simulink model "martin_arbot_v2offset"  (R2020a)
settings: Solver=ode15s  StartTime=0.0  StopTime=15  MaxStep=.01  RelTol=1e-3  AbsTol=1e-4
InitFcn:
  | % currentFolder = pwd;
  | % parent = '../Targeting';
  | % environment = '../Environment';
  | % addpath(genpath(parent));
  | % addpath(genpath(environment));
  | 
  | startup_ARbot;
  | chute2_DataFile;
  | guard_DataFile1;
  | shelf_DataFile1;
  | bin_assembly_DataFile;
values from neighbouring files (symbols this model uses):
  Environment = append(cwd,'/Environment')    [init_root_paths_mac.m]    (also in init_root_paths_windows.m = append(cwd,'\Environment'))
undefined symbols (not defined in the file or in its folder): belt_h, belt_l, belt_spd, belt_w, box1_dim, box2_dim, box3_dim, box4_dim, box5_dim, cube_d, deposit_joint_angle, Extr_Data_LinkHoles, floor_d, floor_l, ikSol, initial_joints, m, n, P_C, safe_via_angles, sigbuilder_block, smiData, X, Y, Z
libraries: sm_lib x145, nesl_utility x78, Contact_Forces_Lib x10, simulink x5, Parts_Lib x5, dspsrcs4 x1
(part 1 of 5)
settings Model: Creator=logan  LastModifiedBy=mcontr
settings SFSimCC: CustomCodeUndefinedFunction=UseInterfaceOnly
settings DiagnosticsConfigSet: SimMechanicsConflictingReferenceFrames=none  SimMechanicsRigidlyBoundBlock=warning

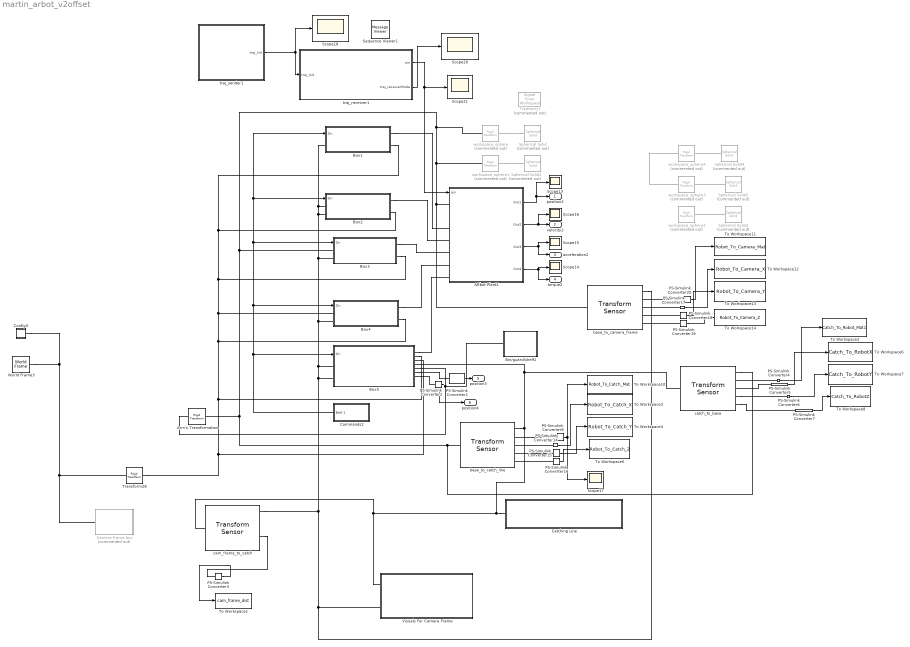
== system martin_arbot_v2offset ==
  ARbot Plant1 : Subsystem
  Arm's Transformation : sm_lib/Frames and Transforms/Rigid Transform  TranslationMethod=Cartesian  TranslationStandardOffset=10  TranslationLengthUnit=m  TranslationStandardAxis=+Y  TranslationCartesianOffset=box_xyz_pos_offset  TranslationROffset=0  TranslationROffsetUnits=m  TranslationZOffset=0  TranslationZOffsetUnits=m  TranslationThetaOffset=0  TranslationThetaOffsetUnits=deg  RotationMethod=RotationSequence  RotationAngleUnits=deg  RotationStandardAxis=+Z  RotationAngle=270  RotationArbitraryAxis=smiData.RigidTransform(1).axis  FollAlignAxisA=+X  BaseAlignAxisA=+Y  FollAlignAxisB=+Y  BaseAlignAxisB=+Z  RotationSequenceAxes=FollowerAxes  RotationSequence=XYZ  RotationSequenceAngles=box_xyz_angle_offset  RotationSequenceAnglesUnits=deg  RotationMatrix=[1 0 0; 0 1 0; 0 0 1]
  Bin/guard/shelf1 : Subsystem
  Box1 : Subsystem
  Box2 : Subsystem
  Box3 : Subsystem
  Box4 : Subsystem
  Box5 : Subsystem
  Camera frame box : Subsystem  Commented=on
  Catching Line : Subsystem
  Commands2 : Subsystem  Tag=STV Subsys  LoadFcn=sigbuilder_block('load');  StartFcn=sigbuilder_block('start');  StopFcn=sigbuilder_block('stop');  ClipboardFcn=sigbuilder_block('clipboard');  mask(Sigbuilder block){tuvar=[0:10]}
      mask help: Simulink:masks:SigbuilderBlock_MD
      mask init:
      | if ~strcmp(get_param(bdroot(gcbh),'SimulationStatus'),'stopped') tuvar = sigbuilder_block('maskInit'); end
      settings: CopyFcn=sigbuilder_block('copy');  DeleteFcn=sigbuilder_block('delete');  ModelCloseFcn=sigbuilder_block('modelClose');  PreSaveFcn=sigbuilder_block('preSave');  PauseFcn=sigbuilder_block('pause');  ContinueFcn=sigbuilder_block('continue');  NameChangeFcn=sigbuilder_block('namechange');  OpenFcn=sigbuilder_block('open',[107 163.5 543 316.5 ]);  CloseFcn=sigbuilder_block('close');
      mask Display: plot(0, 0, 100, 100,[2, 2, 32, 32, 2], [68, 8, 8, 68, 68],[32, 2], [38, 38], [32, 19, 2],[53, 60, 44], [32, 17, 17, 2],[16, 16, 31, 31]);txt = getActiveGroup(gcbh);text(2, 100, txt,'verticalAlignment', 'top');
  Config3 : Subsystem
  PS-Simulink Converter{1..7,9,14..20} (15 alike) : nesl_utility/PS-Simulink Converter  PhysicalDomain=network_engine_domain  SubClassName=ps_output  LeftPortType=input  RightPortType=output  PseudoPeriodic=off  Frequencies=[]  Unit=inherit  AffineConversion=off
  Scope{13..18,20..21} (8 alike) : Scope
  Sequence Viewer1 : MessageViewer
  Spherical Solid : sm_lib/Body Elements/Spherical Solid  Commented=on  GraphicAmbientColor=[0.15 0.15 0.15 1.0]  BasedOnType=Density  CenterOfMass=[0 0 0]  CenterOfMassUnits=m  GraphicDiffuseColor=[1.0 0.6 0.2]  Density=1000  DensityUnits=kg/m^3  DoExposeReferenceFrame=on  GraphicEmissiveColor=[0.0 0.0 0.0 1.0]  ExportEntireGeometry=off  SerializedExposedGeometries=<ExposedGeometries/>  SerializedFrames=<Frames/>  MarkerShape=Sphere  MarkerSize=10  GraphicType=FromGeometry  InertiaType=CalculateFromGeometry  Mass=1  MassUnits=kg  MomentsOfInertia=[1 1 1]  MomentsOfInertiaUnits=kg*m^2  GraphicOpacity=1.0  ProductsOfInertia=[0 0 0]  ProductsOfInertiaUnits=kg*m^2  GraphicShininess=75  GraphicSpecularColor=[0.5 0.5 0.5 1.0]  SphereRadius=0.05  SphereRadiusUnits=m  GraphicVisPropType=SimpleVisualProperties
  Spherical Solid1 : sm_lib/Body Elements/Spherical Solid  Commented=on  GraphicAmbientColor=[0.15 0.15 0.15 1.0]  BasedOnType=Density  CenterOfMass=[0 0 0]  CenterOfMassUnits=m  GraphicDiffuseColor=[1.0 0.6 0.2]  Density=1000  DensityUnits=kg/m^3  DoExposeReferenceFrame=on  GraphicEmissiveColor=[0.0 0.0 0.0 1.0]  ExportEntireGeometry=off  SerializedExposedGeometries=<ExposedGeometries/>  SerializedFrames=<Frames/>  MarkerShape=Sphere  MarkerSize=10  GraphicType=FromGeometry  InertiaType=CalculateFromGeometry  Mass=1  MassUnits=kg  MomentsOfInertia=[1 1 1]  MomentsOfInertiaUnits=kg*m^2  GraphicOpacity=1.0  ProductsOfInertia=[0 0 0]  ProductsOfInertiaUnits=kg*m^2  GraphicShininess=75  GraphicSpecularColor=[0.5 0.5 0.5 1.0]  SphereRadius=0.05  SphereRadiusUnits=m  GraphicVisPropType=SimpleVisualProperties
  Spherical Solid2 : sm_lib/Body Elements/Spherical Solid  Commented=on  GraphicAmbientColor=[0.15 0.15 0.15 1.0]  BasedOnType=Density  CenterOfMass=[0 0 0]  CenterOfMassUnits=m  GraphicDiffuseColor=[0.0 0.8 0.4]  Density=1000  DensityUnits=kg/m^3  DoExposeReferenceFrame=on  GraphicEmissiveColor=[0.0 0.0 0.0 1.0]  ExportEntireGeometry=off  SerializedExposedGeometries=<ExposedGeometries/>  SerializedFrames=<Frames/>  MarkerShape=Sphere  MarkerSize=10  GraphicType=FromGeometry  InertiaType=CalculateFromGeometry  Mass=1  MassUnits=kg  MomentsOfInertia=[1 1 1]  MomentsOfInertiaUnits=kg*m^2  GraphicOpacity=1.0  ProductsOfInertia=[0 0 0]  ProductsOfInertiaUnits=kg*m^2  GraphicShininess=75  GraphicSpecularColor=[0.5 0.5 0.5 1.0]  SphereRadius=0.05  SphereRadiusUnits=m  GraphicVisPropType=SimpleVisualProperties
  Spherical Solid3 : sm_lib/Body Elements/Spherical Solid  Commented=on  GraphicAmbientColor=[0.15 0.15 0.15 1.0]  BasedOnType=Density  CenterOfMass=[0 0 0]  CenterOfMassUnits=m  GraphicDiffuseColor=[0.0 0.8 0.4]  Density=1000  DensityUnits=kg/m^3  DoExposeReferenceFrame=on  GraphicEmissiveColor=[0.0 0.0 0.0 1.0]  ExportEntireGeometry=off  SerializedExposedGeometries=<ExposedGeometries/>  SerializedFrames=<Frames/>  MarkerShape=Sphere  MarkerSize=10  GraphicType=FromGeometry  InertiaType=CalculateFromGeometry  Mass=1  MassUnits=kg  MomentsOfInertia=[1 1 1]  MomentsOfInertiaUnits=kg*m^2  GraphicOpacity=1.0  ProductsOfInertia=[0 0 0]  ProductsOfInertiaUnits=kg*m^2  GraphicShininess=75  GraphicSpecularColor=[0.5 0.5 0.5 1.0]  SphereRadius=0.05  SphereRadiusUnits=m  GraphicVisPropType=SimpleVisualProperties
  Spherical Solid4 : sm_lib/Body Elements/Spherical Solid  Commented=on  GraphicAmbientColor=[0.15 0.15 0.15 1.0]  BasedOnType=Density  CenterOfMass=[0 0 0]  CenterOfMassUnits=m  GraphicDiffuseColor=[0.0 0.8 0.4]  Density=1000  DensityUnits=kg/m^3  DoExposeReferenceFrame=on  GraphicEmissiveColor=[0.0 0.0 0.0 1.0]  ExportEntireGeometry=off  SerializedExposedGeometries=<ExposedGeometries/>  SerializedFrames=<Frames/>  MarkerShape=Sphere  MarkerSize=10  GraphicType=FromGeometry  InertiaType=CalculateFromGeometry  Mass=1  MassUnits=kg  MomentsOfInertia=[1 1 1]  MomentsOfInertiaUnits=kg*m^2  GraphicOpacity=1.0  ProductsOfInertia=[0 0 0]  ProductsOfInertiaUnits=kg*m^2  GraphicShininess=75  GraphicSpecularColor=[0.5 0.5 0.5 1.0]  SphereRadius=0.05  SphereRadiusUnits=m  GraphicVisPropType=SimpleVisualProperties
  To Workspace1 : ToWorkspace  VariableName=cam_frame_dist  SampleTime=-1
      settings: Save2DSignal=2-D array (concatenate along first dimension)
  To Workspace10 : ToWorkspace  VariableName=Robot_To_Catch_Mat  SampleTime=-1
      settings: Save2DSignal=2-D array (concatenate along first dimension)
  To Workspace11 : ToWorkspace  VariableName=Robot_To_Camera_Mat  SampleTime=-1
      settings: Save2DSignal=2-D array (concatenate along first dimension)
  To Workspace12 : ToWorkspace  VariableName=Robot_To_Camera_X  SampleTime=-1
      settings: Save2DSignal=2-D array (concatenate along first dimension)
  To Workspace13 : ToWorkspace  VariableName=Robot_To_Camera_Y  SampleTime=-1
      settings: Save2DSignal=2-D array (concatenate along first dimension)
  To Workspace14 : ToWorkspace  VariableName=Robot_To_Camera_Z  SampleTime=-1
      settings: Save2DSignal=2-D array (concatenate along first dimension)
  To Workspace2 : ToWorkspace  VariableName=Catch_To_Robot_Mat1  SampleTime=-1
      settings: Save2DSignal=2-D array (concatenate along first dimension)
  To Workspace3 : ToWorkspace  VariableName=Robot_To_Catch_X  SampleTime=-1
      settings: Save2DSignal=2-D array (concatenate along first dimension)
  To Workspace4 : ToWorkspace  VariableName=Robot_To_Catch_Y  SampleTime=-1
      settings: Save2DSignal=2-D array (concatenate along first dimension)
  To Workspace5 : ToWorkspace  VariableName=Robot_To_Catch_Z  SampleTime=-1
      settings: Save2DSignal=2-D array (concatenate along first dimension)
  To Workspace6 : ToWorkspace  VariableName=Catch_To_RobotX  SampleTime=-1
      settings: Save2DSignal=2-D array (concatenate along first dimension)
  To Workspace7 : ToWorkspace  VariableName=Catch_To_RobotY  SampleTime=-1
      settings: Save2DSignal=2-D array (concatenate along first dimension)
  To Workspace8 : ToWorkspace  VariableName=Catch_To_RobotZ  SampleTime=-1
      settings: Save2DSignal=2-D array (concatenate along first dimension)
  Trajectory1 : dspsrcs4/Signal From Workspace  Commented=on  X=th  Ts=.08  nsamps=1  OutputAfterFinalValue=Holding final value  ignoreOrWarnInputAndFrameLengths=off  OutputFrames=off
  Transform28 : sm_lib/Frames and Transforms/Rigid Transform  TranslationMethod=Cartesian  TranslationStandardOffset=10  TranslationLengthUnit=m  TranslationStandardAxis=+Y  TranslationCartesianOffset=belt_pos_offset  TranslationROffset=0  TranslationROffsetUnits=m  TranslationZOffset=0  TranslationZOffsetUnits=m  TranslationThetaOffset=0  TranslationThetaOffsetUnits=deg  RotationMethod=RotationSequence  RotationAngleUnits=deg  RotationStandardAxis=+Z  RotationAngle=90  RotationArbitraryAxis=smiData.RigidTransform(1).axis  FollAlignAxisA=+X  BaseAlignAxisA=+Y  FollAlignAxisB=+Y  BaseAlignAxisB=+Z  RotationSequenceAxes=BaseAxes  RotationSequence=XYZ  RotationSequenceAngles=belt_angle_offset  RotationSequenceAnglesUnits=deg  RotationMatrix=[1 0 0; 0 1 0; 0 0 1]
  Visuals For Camera Frame : Subsystem
  World Frame3 : sm_lib/Frames and Transforms/World Frame
  base_to_camera_frame : sm_lib/Frames and Transforms/Transform Sensor  MeasurementFrame=Base  SenseAngle=off  SenseAxis=off  SenseAngle1=off  SenseAngle2=off  SenseAngle3=off  SenseQ=off  SenseR=on  SenseOmegaX=off  SenseOmegaY=off  SenseOmegaZ=off  SenseOmega1=off  SenseOmega2=off  SenseOmega3=off  SenseQDot=off  SenseRDot=off  SenseAlphaX=off  SenseAlphaY=off  SenseAlphaZ=off  SenseAlpha1=off  SenseAlpha2=off  SenseAlpha3=off  SenseQDDot=off  SenseRDDot=off  SenseX=on  SenseY=on  SenseZ=on  SenseRad=off  SenseAzim=off  SenseDist=off  SenseInc=off  SenseXDot=off  SenseYDot=off  SenseZDot=off  SenseRadDot=off  SenseAzimDot=off  SenseDistDot=off  SenseIncDot=off  SenseXDDot=off  SenseYDDot=off  SenseZDDot=off  SenseRadDDot=off  SenseAzimDDot=off  SenseDistDDot=off  SenseIncDDot=off
  base_to_catch_line : sm_lib/Frames and Transforms/Transform Sensor  MeasurementFrame=Base  SenseAngle=off  SenseAxis=off  SenseAngle1=off  SenseAngle2=off  SenseAngle3=off  SenseQ=off  SenseR=on  SenseOmegaX=off  SenseOmegaY=off  SenseOmegaZ=off  SenseOmega1=off  SenseOmega2=off  SenseOmega3=off  SenseQDot=off  SenseRDot=off  SenseAlphaX=off  SenseAlphaY=off  SenseAlphaZ=off  SenseAlpha1=off  SenseAlpha2=off  SenseAlpha3=off  SenseQDDot=off  SenseRDDot=off  SenseX=on  SenseY=on  SenseZ=on  SenseRad=off  SenseAzim=off  SenseDist=off  SenseInc=off  SenseXDot=off  SenseYDot=off  SenseZDot=off  SenseRadDot=off  SenseAzimDot=off  SenseDistDot=off  SenseIncDot=off  SenseXDDot=off  SenseYDDot=off  SenseZDDot=off  SenseRadDDot=off  SenseAzimDDot=off  SenseDistDDot=off  SenseIncDDot=off
  cam_frame_to_catch : sm_lib/Frames and Transforms/Transform Sensor  MeasurementFrame=Base  SenseAngle=off  SenseAxis=off  SenseAngle1=off  SenseAngle2=off  SenseAngle3=off  SenseQ=off  SenseR=on  SenseOmegaX=off  SenseOmegaY=off  SenseOmegaZ=off  SenseOmega1=off  SenseOmega2=off  SenseOmega3=off  SenseQDot=off  SenseRDot=off  SenseAlphaX=off  SenseAlphaY=off  SenseAlphaZ=off  SenseAlpha1=off  SenseAlpha2=off  SenseAlpha3=off  SenseQDDot=off  SenseRDDot=off  SenseX=on  SenseY=on  SenseZ=on  SenseRad=off  SenseAzim=off  SenseDist=off  SenseInc=off  SenseXDot=off  SenseYDot=off  SenseZDot=off  SenseRadDot=off  SenseAzimDot=off  SenseDistDot=off  SenseIncDot=off  SenseXDDot=off  SenseYDDot=off  SenseZDDot=off  SenseRadDDot=off  SenseAzimDDot=off  SenseDistDDot=off  SenseIncDDot=off
  catch_to_base : sm_lib/Frames and Transforms/Transform Sensor  MeasurementFrame=Base  SenseAngle=off  SenseAxis=off  SenseAngle1=off  SenseAngle2=off  SenseAngle3=off  SenseQ=off  SenseR=on  SenseOmegaX=off  SenseOmegaY=off  SenseOmegaZ=off  SenseOmega1=off  SenseOmega2=off  SenseOmega3=off  SenseQDot=off  SenseRDot=off  SenseAlphaX=off  SenseAlphaY=off  SenseAlphaZ=off  SenseAlpha1=off  SenseAlpha2=off  SenseAlpha3=off  SenseQDDot=off  SenseRDDot=off  SenseX=on  SenseY=on  SenseZ=on  SenseRad=off  SenseAzim=off  SenseDist=off  SenseInc=off  SenseXDot=off  SenseYDot=off  SenseZDot=off  SenseRadDot=off  SenseAzimDot=off  SenseDistDot=off  SenseIncDot=off  SenseXDDot=off  SenseYDDot=off  SenseZDDot=off  SenseRadDDot=off  SenseAzimDDot=off  SenseDistDDot=off  SenseIncDDot=off
  traj_receiver1 : Stateflow chart  TreatAsAtomicUnit=on
  traj_sender1 : Stateflow chart  TreatAsAtomicUnit=on
  workspace_sphere : sm_lib/Frames and Transforms/Rigid Transform  Commented=on  TranslationMethod=Cartesian  TranslationStandardOffset=10  TranslationLengthUnit=m  TranslationStandardAxis=+Y  TranslationCartesianOffset=Arc_Midpoint  TranslationROffset=0  TranslationROffsetUnits=m  TranslationZOffset=0  TranslationZOffsetUnits=m  TranslationThetaOffset=0  TranslationThetaOffsetUnits=deg  RotationMethod=RotationMatrix  RotationAngleUnits=deg  RotationStandardAxis=+Z  RotationAngle=270  RotationArbitraryAxis=smiData.RigidTransform(1).axis  FollAlignAxisA=+X  BaseAlignAxisA=+Y  FollAlignAxisB=+Y  BaseAlignAxisB=+Z  RotationSequenceAxes=FollowerAxes  RotationSequence=XYZ  RotationSequenceAngles=box_xyz_angle_offset  RotationSequenceAnglesUnits=deg  RotationMatrix=robot_base_to_camera_frame_rot
  workspace_sphere1 : sm_lib/Frames and Transforms/Rigid Transform  Commented=on  TranslationMethod=Cartesian  TranslationStandardOffset=10  TranslationLengthUnit=m  TranslationStandardAxis=+Y  TranslationCartesianOffset=Arc_Start  TranslationROffset=0  TranslationROffsetUnits=m  TranslationZOffset=0  TranslationZOffsetUnits=m  TranslationThetaOffset=0  TranslationThetaOffsetUnits=deg  RotationMethod=RotationMatrix  RotationAngleUnits=deg  RotationStandardAxis=+Z  RotationAngle=270  RotationArbitraryAxis=smiData.RigidTransform(1).axis  FollAlignAxisA=+X  BaseAlignAxisA=+Y  FollAlignAxisB=+Y  BaseAlignAxisB=+Z  RotationSequenceAxes=FollowerAxes  RotationSequence=XYZ  RotationSequenceAngles=box_xyz_angle_offset  RotationSequenceAnglesUnits=deg  RotationMatrix=robot_base_to_camera_frame_rot
  workspace_sphere2 : sm_lib/Frames and Transforms/Rigid Transform  Commented=on  TranslationMethod=Cartesian  TranslationStandardOffset=10  TranslationLengthUnit=m  TranslationStandardAxis=+Y  TranslationCartesianOffset=P_C(1,1:3)  TranslationROffset=0  TranslationROffsetUnits=m  TranslationZOffset=0  TranslationZOffsetUnits=m  TranslationThetaOffset=0  TranslationThetaOffsetUnits=deg  RotationMethod=None  RotationAngleUnits=deg  RotationStandardAxis=+Z  RotationAngle=270  RotationArbitraryAxis=smiData.RigidTransform(1).axis  FollAlignAxisA=+X  BaseAlignAxisA=+Y  FollAlignAxisB=+Y  BaseAlignAxisB=+Z  RotationSequenceAxes=FollowerAxes  RotationSequence=XYZ  RotationSequenceAngles=box_xyz_angle_offset  RotationSequenceAnglesUnits=deg  RotationMatrix=robot_base_to_camera_frame_rot
  workspace_sphere3 : sm_lib/Frames and Transforms/Rigid Transform  Commented=on  TranslationMethod=Cartesian  TranslationStandardOffset=10  TranslationLengthUnit=m  TranslationStandardAxis=+Y  TranslationCartesianOffset=P_C(2,1:3)  TranslationROffset=0  TranslationROffsetUnits=m  TranslationZOffset=0  TranslationZOffsetUnits=m  TranslationThetaOffset=0  TranslationThetaOffsetUnits=deg  RotationMethod=None  RotationAngleUnits=deg  RotationStandardAxis=+Z  RotationAngle=270  RotationArbitraryAxis=smiData.RigidTransform(1).axis  FollAlignAxisA=+X  BaseAlignAxisA=+Y  FollAlignAxisB=+Y  BaseAlignAxisB=+Z  RotationSequenceAxes=FollowerAxes  RotationSequence=XYZ  RotationSequenceAngles=box_xyz_angle_offset  RotationSequenceAnglesUnits=deg  RotationMatrix=robot_base_to_camera_frame_rot
  workspace_sphere4 : sm_lib/Frames and Transforms/Rigid Transform  Commented=on  TranslationMethod=Cartesian  TranslationStandardOffset=10  TranslationLengthUnit=m  TranslationStandardAxis=+Y  TranslationCartesianOffset=P_C(3,1:3)  TranslationROffset=0  TranslationROffsetUnits=m  TranslationZOffset=0  TranslationZOffsetUnits=m  TranslationThetaOffset=0  TranslationThetaOffsetUnits=deg  RotationMethod=None  RotationAngleUnits=deg  RotationStandardAxis=+Z  RotationAngle=270  RotationArbitraryAxis=smiData.RigidTransform(1).axis  FollAlignAxisA=+X  BaseAlignAxisA=+Y  FollAlignAxisB=+Y  BaseAlignAxisB=+Z  RotationSequenceAxes=FollowerAxes  RotationSequence=XYZ  RotationSequenceAngles=box_xyz_angle_offset  RotationSequenceAnglesUnits=deg  RotationMatrix=robot_base_to_camera_frame_rot
  position2 : Outport  VectorParamsAs1DForOutWhenUnconnected=off
  velocity2 : Outport  Port=2  VectorParamsAs1DForOutWhenUnconnected=off
  acceleration2 : Outport  Port=3  VectorParamsAs1DForOutWhenUnconnected=off
  torque2 : Outport  Port=4  VectorParamsAs1DForOutWhenUnconnected=off
  position3 : Outport  Port=5  Unit=rad/s  VectorParamsAs1DForOutWhenUnconnected=off
  position4 : Outport  Port=6  VectorParamsAs1DForOutWhenUnconnected=off
  wires:
  PS-Simulink Converter2/1 -> position4/1
  ARbot Plant1/4(Out4) -> Scope14/1, torque2/1
  PS-Simulink Converter15/1 -> To Workspace4/1
  traj_receiver1/1(qin) -> Scope21/1, ARbot Plant1/1(qin)
  ARbot Plant1/1(Out1) -> Scope13/1, position2/1
  PS-Simulink Converter14/1 -> To Workspace3/1
  Commands2/1(Belt 1) -> Box4/1(On), Box3/1(On), Box1/1(On), Box2/1(On), Box5/1(On)
  ARbot Plant1/3(Out3) -> Scope15/1, acceleration2/1
  ARbot Plant1/2(Out2) -> Scope16/1, velocity2/1
  PS-Simulink Converter9/1 -> To Workspace10/1, Scope17/1
  PS-Simulink Converter16/1 -> To Workspace5/1
  PS-Simulink Converter1/1 -> position3/1
  traj_sender1/1(traj_Init) -> traj_receiver1/1(traj_Init), Scope18/1
  PS-Simulink Converter18/1 -> To Workspace13/1
  PS-Simulink Converter19/1 -> To Workspace14/1
  PS-Simulink Converter20/1 -> To Workspace11/1
  PS-Simulink Converter17/1 -> To Workspace12/1
  PS-Simulink Converter3/1 -> To Workspace1/1
  PS-Simulink Converter4/1 -> To Workspace2/1
  PS-Simulink Converter5/1 -> To Workspace6/1
  PS-Simulink Converter6/1 -> To Workspace7/1
  PS-Simulink Converter7/1 -> To Workspace8/1
  traj_receiver1/2(traj_receiverMode) -> Scope20/1
  connections:
  Box4/LConn2 -- Box3/LConn2 -- Box1/LConn1 -- Box2/LConn1 -- Box2/LConn2 -- Box5/LConn1 -- cam_frame_to_catch/RConn1 -- base_to_camera_frame/RConn1 -- Visuals For Camera Frame/LConn2 -- Box5/LConn2
  Box5/RConn5 -- Bin/guard/shelf1/LConn1 -- Arm's Transformation/LConn1
  Box2/RConn2 -- Box1/RConn2 -- Box5/RConn3 -- Transform28/RConn1 -- Box5/RConn2 -- Box4/RConn2 -- Box4/LConn1 -- Box3/RConn2
  World Frame3/RConn1 -- Transform28/LConn1 -- Camera frame box/LConn1 -- Config3/RConn1
  Box3/LConn1 -- base_to_camera_frame/LConn1 -- ARbot Plant1/LConn1 -- workspace_sphere1/LConn1 -- workspace_sphere/LConn1 -- base_to_catch_line/LConn1 -- catch_to_base/RConn1 -- Arm's Transformation/RConn1
  Box4/RConn1 -- ARbot Plant1/LConn6
  Box5/RConn6 -- PS-Simulink Converter1/LConn1
  PS-Simulink Converter16/LConn1 -- base_to_catch_line/RConn5
  PS-Simulink Converter2/LConn1 -- Box5/RConn7
  PS-Simulink Converter14/LConn1 -- base_to_catch_line/RConn3
  PS-Simulink Converter9/LConn1 -- base_to_catch_line/RConn2
  Box3/RConn1 -- ARbot Plant1/LConn5
  Box1/RConn1 -- ARbot Plant1/LConn3
  Catching Line/LConn1 -- cam_frame_to_catch/LConn1 -- Visuals For Camera Frame/LConn1 -- base_to_catch_line/RConn1 -- catch_to_base/LConn1 -- Box5/RConn4
  Box5/RConn1 -- ARbot Plant1/LConn7
  PS-Simulink Converter15/LConn1 -- base_to_catch_line/RConn4
  Box2/RConn1 -- ARbot Plant1/LConn4
  PS-Simulink Converter20/LConn1 -- base_to_camera_frame/RConn2
  PS-Simulink Converter18/LConn1 -- base_to_camera_frame/RConn4
  PS-Simulink Converter19/LConn1 -- base_to_camera_frame/RConn5
  PS-Simulink Converter17/LConn1 -- base_to_camera_frame/RConn3
  cam_frame_to_catch/RConn4 -- PS-Simulink Converter3/LConn1
  PS-Simulink Converter4/LConn1 -- catch_to_base/RConn2
  PS-Simulink Converter5/LConn1 -- catch_to_base/RConn3
  catch_to_base/RConn4 -- PS-Simulink Converter6/LConn1
  catch_to_base/RConn5 -- PS-Simulink Converter7/LConn1
  workspace_sphere/RConn1 -- Spherical Solid/RConn1
  workspace_sphere1/RConn1 -- Spherical Solid1/RConn1
  Spherical Solid3/RConn1 -- workspace_sphere2/RConn1
  Spherical Solid2/RConn1 -- workspace_sphere3/RConn1
  workspace_sphere4/RConn1 -- Spherical Solid4/RConn1
  workspace_sphere3/LConn1 -- workspace_sphere4/LConn1

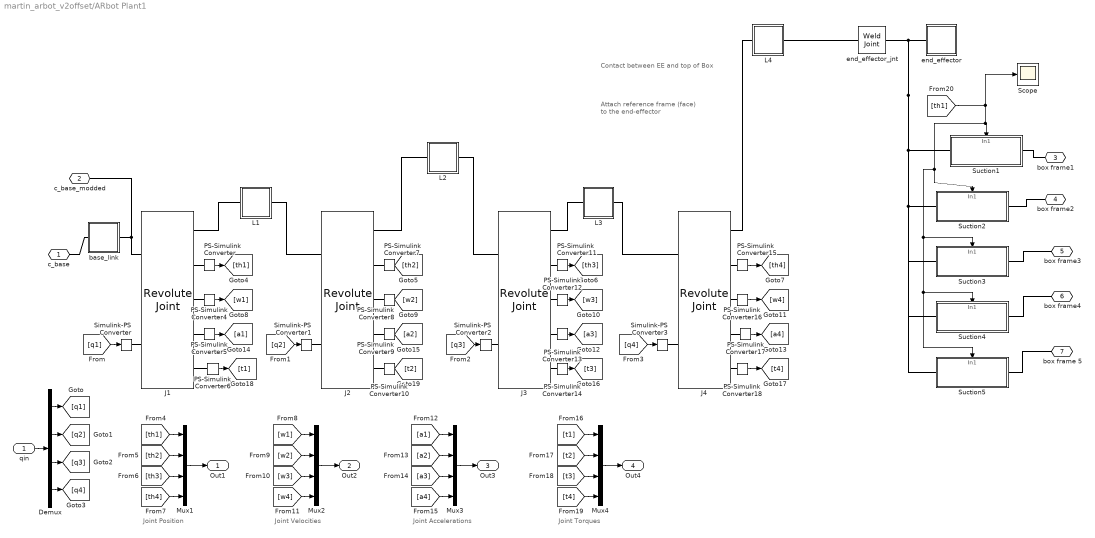
== system martin_arbot_v2offset/ARbot Plant1 ==
  note: Contact between EE and top
      | of Box
  note: Joint Position
  note: Joint Velocities
  note: Joint Accelerations
  note: Joint Torques
  note: Attach reference frame (face)
      | to the end-effector
  qin : Inport
  Demux : Demux
  J{1..4} (4 alike) : sm_lib/Joints/Revolute Joint  JointMode=Normal  SenseConstraintForce=off  SenseConstraintForceX=off  SenseConstraintForceY=off  SenseConstraintForceZ=off  SenseConstraintTorque=off  SenseConstraintTorqueX=off  SenseConstraintTorqueY=off  SenseConstraintTorqueZ=off  SenseTotalForce=off  SenseTotalForceX=off  SenseTotalForceY=off  SenseTotalForceZ=off  SenseTotalTorque=off  SenseTotalTorqueX=off  SenseTotalTorqueY=off  SenseTotalTorqueZ=off  CompositeWrenchDir=FollowerOnBase  CompositeWrenchFrame=BaseFrame  EquilibriumPosition=0  EquilibriumPositionUnits=deg  SpringStiffness=0  SpringStiffnessUnits=N*m/deg  DampingCoefficient=0  DampingCoefficientUnits=m^2*kg/s/rad  TorqueActuationMode=ComputedTorque  MotionActuationMode=InputMotion  SensePosition=on  SenseVelocity=on  SenseAcceleration=on  SenseTorqueForce=on  SenseLowerLimitTorqueForce=off  SenseUpperLimitTorqueForce=off  LowerLimitSpecify=off  LowerLimitBound=-90  LowerLimitBoundUnits=deg  LowerLimitStiffness=1e4  LowerLimitStiffnessUnits=N*m/deg  LowerLimitDamping=10  LowerLimitDampingUnits=N*m/(deg/s)  LowerLimitTransitionRegionWidth=0.1  LowerLimitTransitionRegionWidthUnits=deg  UpperLimitSpecify=off  UpperLimitBound=90  UpperLimitBoundUnits=deg  UpperLimitStiffness=1e4  UpperLimitStiffnessUnits=N*m/deg  UpperLimitDamping=10  UpperLimitDampingUnits=N*m/(deg/s)  UpperLimitTransitionRegionWidth=0.1  UpperLimitTransitionRegionWidthUnits=deg  PositionTargetSpecify=off  PositionTargetPriority=High  PositionTargetValue=0  PositionTargetValueUnits=deg  VelocityTargetSpecify=off  VelocityTargetPriority=High  VelocityTargetValue=0  VelocityTargetValueUnits=deg/s
  L1 : Subsystem
  L2 : Subsystem
  L3 : Subsystem
  L4 : Subsystem
  Mux{1..4} (4 alike) : Mux
  PS-Simulink Converter{,4..5,7..9,11..13,15..17} (12 alike) : nesl_utility/PS-Simulink Converter  PhysicalDomain=network_engine_domain  SubClassName=ps_output  LeftPortType=input  RightPortType=output  PseudoPeriodic=off  Frequencies=[]  Unit=1  AffineConversion=off
  PS-Simulink Converter{6,10,14,18} (4 alike) : nesl_utility/PS-Simulink Converter  PhysicalDomain=network_engine_domain  SubClassName=ps_output  LeftPortType=input  RightPortType=output  PseudoPeriodic=off  Frequencies=[]  Unit=N*m  AffineConversion=off
  Scope : Scope
  Simulink-PS Converter : nesl_utility/Simulink-PS Converter  PhysicalDomain=network_engine_domain  SubClassName=ps_input  LeftPortType=input  RightPortType=output  PseudoPeriodic=off  Frequencies=[]  NoiseDistribution=none  NoiseParameters=[]  Unit=rad  AffineConversion=off  FilteringAndDerivatives=filter  SimscapeFilterOrder=2  InputFilterTimeConstant=0.01  UdotUserProvided=0
  Simulink-PS Converter1 : nesl_utility/Simulink-PS Converter  PhysicalDomain=network_engine_domain  SubClassName=ps_input  LeftPortType=input  RightPortType=output  PseudoPeriodic=off  Frequencies=[]  NoiseDistribution=none  NoiseParameters=[]  Unit=rad  AffineConversion=off  FilteringAndDerivatives=filter  SimscapeFilterOrder=2  InputFilterTimeConstant=.01  UdotUserProvided=0
  Simulink-PS Converter2 : nesl_utility/Simulink-PS Converter  PhysicalDomain=network_engine_domain  SubClassName=ps_input  LeftPortType=input  RightPortType=output  PseudoPeriodic=off  Frequencies=[]  NoiseDistribution=none  NoiseParameters=[]  Unit=rad  AffineConversion=off  FilteringAndDerivatives=filter  SimscapeFilterOrder=2  InputFilterTimeConstant=0.01  UdotUserProvided=0
  Simulink-PS Converter3 : nesl_utility/Simulink-PS Converter  PhysicalDomain=network_engine_domain  SubClassName=ps_input  LeftPortType=input  RightPortType=output  PseudoPeriodic=off  Frequencies=[]  NoiseDistribution=none  NoiseParameters=[]  Unit=rad  AffineConversion=off  FilteringAndDerivatives=filter  SimscapeFilterOrder=2  InputFilterTimeConstant=0.01  UdotUserProvided=0
  Suction1 : Subsystem
      settings: PortSchema="{\"entries\":[{\"content\":{\"sides\":[{\"content\":{\"connectorIds\":[\"LConn1\"]},\"type\":\"ConnectorPlacement.EquallySpacedRectSide\",\"uuid\":\"79633fc7-8505-43b1-81c2-e32c3764fd2a\"},{\"content\":{\"connectorIds\":[\"RConn1\"],\"side\":\"RIGHT\"},\"type\":\"ConnectorPlacement.EquallySpacedRectSide\",\"uuid\":\"2fbeebe5-d9a4-4c9f-83da-18d8f5f7a16b\"},{\"content\":{\"connectorIds\":[\"In1\"],\"side\":\"TOP\"},\"type\":\"ConnectorPlacement.EquallySpacedRectSide\",\"uuid\":\"e7fe1fa9-bd94-4e7e-b745-4e3da324ca91\"}]},\"type\":\"ConnectorPlacement.EquallySpacedConnector\",\"uuid\":\"68ee8142-98d6-402d-88d0-44e443221a72\"}],\"packageUris\":[\"http://schema.mathworks.com/mf0/Connector/19700101\"],\"version\":\"1.0\"}"
  Suction2 : Subsystem
      settings: PortSchema="{\"entries\":[{\"content\":{\"sides\":[{\"content\":{\"connectorIds\":[\"LConn1\"]},\"type\":\"ConnectorPlacement.EquallySpacedRectSide\",\"uuid\":\"79633fc7-8505-43b1-81c2-e32c3764fd2a\"},{\"content\":{\"connectorIds\":[\"RConn1\"],\"side\":\"RIGHT\"},\"type\":\"ConnectorPlacement.EquallySpacedRectSide\",\"uuid\":\"2fbeebe5-d9a4-4c9f-83da-18d8f5f7a16b\"},{\"content\":{\"connectorIds\":[\"In1\"],\"side\":\"TOP\"},\"type\":\"ConnectorPlacement.EquallySpacedRectSide\",\"uuid\":\"e7fe1fa9-bd94-4e7e-b745-4e3da324ca91\"}]},\"type\":\"ConnectorPlacement.EquallySpacedConnector\",\"uuid\":\"68ee8142-98d6-402d-88d0-44e443221a72\"}],\"packageUris\":[\"http://schema.mathworks.com/mf0/Connector/19700101\"],\"version\":\"1.0\"}"
  Suction3 : Subsystem
      settings: PortSchema="{\"entries\":[{\"content\":{\"sides\":[{\"content\":{\"connectorIds\":[\"LConn1\"]},\"type\":\"ConnectorPlacement.EquallySpacedRectSide\",\"uuid\":\"79633fc7-8505-43b1-81c2-e32c3764fd2a\"},{\"content\":{\"connectorIds\":[\"RConn1\"],\"side\":\"RIGHT\"},\"type\":\"ConnectorPlacement.EquallySpacedRectSide\",\"uuid\":\"2fbeebe5-d9a4-4c9f-83da-18d8f5f7a16b\"},{\"content\":{\"connectorIds\":[\"In1\"],\"side\":\"TOP\"},\"type\":\"ConnectorPlacement.EquallySpacedRectSide\",\"uuid\":\"e7fe1fa9-bd94-4e7e-b745-4e3da324ca91\"}]},\"type\":\"ConnectorPlacement.EquallySpacedConnector\",\"uuid\":\"68ee8142-98d6-402d-88d0-44e443221a72\"}],\"packageUris\":[\"http://schema.mathworks.com/mf0/Connector/19700101\"],\"version\":\"1.0\"}"
  Suction4 : Subsystem
      settings: PortSchema="{\"entries\":[{\"content\":{\"sides\":[{\"content\":{\"connectorIds\":[\"LConn1\"]},\"type\":\"ConnectorPlacement.EquallySpacedRectSide\",\"uuid\":\"79633fc7-8505-43b1-81c2-e32c3764fd2a\"},{\"content\":{\"connectorIds\":[\"RConn1\"],\"side\":\"RIGHT\"},\"type\":\"ConnectorPlacement.EquallySpacedRectSide\",\"uuid\":\"2fbeebe5-d9a4-4c9f-83da-18d8f5f7a16b\"},{\"content\":{\"connectorIds\":[\"In1\"],\"side\":\"TOP\"},\"type\":\"ConnectorPlacement.EquallySpacedRectSide\",\"uuid\":\"e7fe1fa9-bd94-4e7e-b745-4e3da324ca91\"}]},\"type\":\"ConnectorPlacement.EquallySpacedConnector\",\"uuid\":\"68ee8142-98d6-402d-88d0-44e443221a72\"}],\"packageUris\":[\"http://schema.mathworks.com/mf0/Connector/19700101\"],\"version\":\"1.0\"}"
  Suction5 : Subsystem
      settings: PortSchema="{\"entries\":[{\"content\":{\"sides\":[{\"content\":{\"connectorIds\":[\"LConn1\"]},\"type\":\"ConnectorPlacement.EquallySpacedRectSide\",\"uuid\":\"79633fc7-8505-43b1-81c2-e32c3764fd2a\"},{\"content\":{\"connectorIds\":[\"RConn1\"],\"side\":\"RIGHT\"},\"type\":\"ConnectorPlacement.EquallySpacedRectSide\",\"uuid\":\"2fbeebe5-d9a4-4c9f-83da-18d8f5f7a16b\"},{\"content\":{\"connectorIds\":[\"In1\"],\"side\":\"TOP\"},\"type\":\"ConnectorPlacement.EquallySpacedRectSide\",\"uuid\":\"e7fe1fa9-bd94-4e7e-b745-4e3da324ca91\"}]},\"type\":\"ConnectorPlacement.EquallySpacedConnector\",\"uuid\":\"68ee8142-98d6-402d-88d0-44e443221a72\"}],\"packageUris\":[\"http://schema.mathworks.com/mf0/Connector/19700101\"],\"version\":\"1.0\"}"
  base_link : Subsystem
  end_effector : Subsystem
  end_effector_jnt : sm_lib/Joints/Weld Joint  JointMode=Normal  SenseConstraintForce=off  SenseConstraintForceX=off  SenseConstraintForceY=off  SenseConstraintForceZ=off  SenseConstraintTorque=off  SenseConstraintTorqueX=off  SenseConstraintTorqueY=off  SenseConstraintTorqueZ=off  SenseTotalForce=off  SenseTotalForceX=off  SenseTotalForceY=off  SenseTotalForceZ=off  SenseTotalTorque=off  SenseTotalTorqueX=off  SenseTotalTorqueY=off  SenseTotalTorqueZ=off  CompositeWrenchDir=FollowerOnBase  CompositeWrenchFrame=BaseFrame
  c_base : PMIOPort  Side=Left
  c_base_modded : PMIOPort  Port=2  Side=Left
  box frame1 : PMIOPort  Port=3  Side=Left
  box frame2 : PMIOPort  Port=4  Side=Left
  box frame3 : PMIOPort  Port=5  Side=Left
  box frame4 : PMIOPort  Port=6  Side=Left
  box frame 5 : PMIOPort  Port=7  Side=Left
  Out1 : Outport  VectorParamsAs1DForOutWhenUnconnected=off
  Out2 : Outport  Port=2  VectorParamsAs1DForOutWhenUnconnected=off
  Out3 : Outport  Port=3  VectorParamsAs1DForOutWhenUnconnected=off
  Out4 : Outport  Port=4  VectorParamsAs1DForOutWhenUnconnected=off
  wires:
  PS-Simulink Converter18/1 -> [t4]
  PS-Simulink Converter16/1 -> [w4]
  [t4] -> Mux4/4
  PS-Simulink Converter/1 -> [th1]
  PS-Simulink Converter13/1 -> [a3]
  PS-Simulink Converter11/1 -> [th3]
  [t3] -> Mux4/3
  PS-Simulink Converter6/1 -> [t1]
  PS-Simulink Converter5/1 -> [a1]
  Mux4/1 -> Out4/1
  Mux3/1 -> Out3/1
  PS-Simulink Converter4/1 -> [w1]
  [q4] -> Simulink-PS Converter3/1
  [a2] -> Mux3/2
  PS-Simulink Converter10/1 -> [t2]
  Demux/1 -> [q1]
  [q1] -> Simulink-PS Converter/1
  PS-Simulink Converter12/1 -> [w3]
  [t1] -> Mux4/1
  [a3] -> Mux3/3
  [t2] -> Mux4/2
  [th1] -> Mux1/1
  PS-Simulink Converter7/1 -> [th2]
  [a4] -> Mux3/4
  [a1] -> Mux3/1
  [w1] -> Mux2/1
  [th4] -> Mux1/4
  [th2] -> Mux1/2
  Demux/3 -> [q3]
  [th3] -> Mux1/3
  PS-Simulink Converter14/1 -> [t3]
  Demux/4 -> [q4]
  Demux/2 -> [q2]
  PS-Simulink Converter9/1 -> [a2]
  Mux1/1 -> Out1/1
  qin/1 -> Demux/1
  Mux2/1 -> Out2/1
  PS-Simulink Converter15/1 -> [th4]
  PS-Simulink Converter17/1 -> [a4]
  PS-Simulink Converter8/1 -> [w2]
  [q2] -> Simulink-PS Converter1/1
  [q3] -> Simulink-PS Converter2/1
  [w3] -> Mux2/3
  [w4] -> Mux2/4
  [w2] -> Mux2/2
  [th1] -> Scope/1, Suction1/1(In1), Suction5/1(In1), Suction4/1(In1), Suction3/1(In1), Suction2/1(In1)
  connections:
  J3/RConn1 -- L3/LConn1
  Simulink-PS Converter3/RConn1 -- J4/LConn2
  J1/LConn1 -- base_link/RConn1 -- c_base_modded/RConn1
  J1/RConn1 -- L1/LConn1
  J2/LConn1 -- L1/RConn1
  J2/RConn1 -- L2/LConn1
  J3/LConn1 -- L2/RConn1
  J2/RConn2 -- PS-Simulink Converter7/LConn1
  J4/LConn1 -- L3/RConn1
  J3/RConn3 -- PS-Simulink Converter12/LConn1
  PS-Simulink Converter18/LConn1 -- J4/RConn5
  Simulink-PS Converter1/RConn1 -- J2/LConn2
  PS-Simulink Converter4/LConn1 -- J1/RConn3
  J3/RConn5 -- PS-Simulink Converter14/LConn1
  J3/RConn4 -- PS-Simulink Converter13/LConn1
  J4/RConn4 -- PS-Simulink Converter17/LConn1
  PS-Simulink Converter11/LConn1 -- J3/RConn2
  J4/RConn3 -- PS-Simulink Converter16/LConn1
  J2/RConn4 -- PS-Simulink Converter9/LConn1
  J2/RConn5 -- PS-Simulink Converter10/LConn1
  PS-Simulink Converter8/LConn1 -- J2/RConn3
  PS-Simulink Converter15/LConn1 -- J4/RConn2
  Simulink-PS Converter2/RConn1 -- J3/LConn2
  J1/RConn2 -- PS-Simulink Converter/LConn1
  PS-Simulink Converter6/LConn1 -- J1/RConn5
  J1/RConn4 -- PS-Simulink Converter5/LConn1
  c_base/RConn1 -- base_link/LConn1
  Simulink-PS Converter/RConn1 -- J1/LConn2
  L4/RConn1 -- end_effector_jnt/LConn1
  J4/RConn1 -- L4/LConn1
  end_effector/LConn1 -- Suction5/LConn1 -- Suction4/LConn1 -- Suction3/LConn1 -- Suction2/LConn1 -- Suction1/LConn1 -- end_effector_jnt/RConn1
  Suction1/RConn1 -- box frame1/RConn1
  Suction2/RConn1 -- box frame2/RConn1
  Suction3/RConn1 -- box frame3/RConn1
  Suction4/RConn1 -- box frame4/RConn1
  Suction5/RConn1 -- box frame 5/RConn1

== system martin_arbot_v2offset/Bin//guard//shelf1 ==
  Transform2 : sm_lib/Frames and Transforms/Rigid Transform  TranslationMethod=Cartesian  TranslationStandardOffset=10  TranslationLengthUnit=m  TranslationStandardAxis=+Y  TranslationCartesianOffset=guard1_pos_offset  TranslationROffset=0  TranslationROffsetUnits=m  TranslationZOffset=0  TranslationZOffsetUnits=m  TranslationThetaOffset=0  TranslationThetaOffsetUnits=deg  RotationMethod=RotationSequence  RotationAngleUnits=deg  RotationStandardAxis=+Z  RotationAngle=90  RotationArbitraryAxis=smiData.RigidTransform(1).axis  FollAlignAxisA=+X  BaseAlignAxisA=+Y  FollAlignAxisB=+Y  BaseAlignAxisB=+Z  RotationSequenceAxes=BaseAxes  RotationSequence=XYZ  RotationSequenceAngles=guard1_angle_offset  RotationSequenceAnglesUnits=deg  RotationMatrix=[1 0 0; 0 1 0; 0 0 1]
  Transform3 : sm_lib/Frames and Transforms/Rigid Transform  TranslationMethod=Cartesian  TranslationStandardOffset=10  TranslationLengthUnit=m  TranslationStandardAxis=+Y  TranslationCartesianOffset=guard2_pos_offset  TranslationROffset=0  TranslationROffsetUnits=m  TranslationZOffset=0  TranslationZOffsetUnits=m  TranslationThetaOffset=0  TranslationThetaOffsetUnits=deg  RotationMethod=RotationSequence  RotationAngleUnits=deg  RotationStandardAxis=+Z  RotationAngle=90  RotationArbitraryAxis=smiData.RigidTransform(1).axis  FollAlignAxisA=+X  BaseAlignAxisA=+Y  FollAlignAxisB=+Y  BaseAlignAxisB=+Z  RotationSequenceAxes=BaseAxes  RotationSequence=XYZ  RotationSequenceAngles=guard2_angle_offset  RotationSequenceAnglesUnits=deg  RotationMatrix=[1 0 0; 0 1 0; 0 0 1]
  Transform34 : sm_lib/Frames and Transforms/Rigid Transform  TranslationMethod=Cartesian  TranslationStandardOffset=10  TranslationLengthUnit=m  TranslationStandardAxis=+Y  TranslationCartesianOffset=shelf_pos_offset  TranslationROffset=0  TranslationROffsetUnits=m  TranslationZOffset=0  TranslationZOffsetUnits=m  TranslationThetaOffset=0  TranslationThetaOffsetUnits=deg  RotationMethod=RotationSequence  RotationAngleUnits=deg  RotationStandardAxis=+Z  RotationAngle=90  RotationArbitraryAxis=smiData.RigidTransform(1).axis  FollAlignAxisA=+X  BaseAlignAxisA=+Y  FollAlignAxisB=+Y  BaseAlignAxisB=+Z  RotationSequenceAxes=BaseAxes  RotationSequence=XYZ  RotationSequenceAngles=shelf_angle_offset  RotationSequenceAnglesUnits=deg  RotationMatrix=[1 0 0; 0 1 0; 0 0 1]
  Transform4 : sm_lib/Frames and Transforms/Rigid Transform  Commented=on  TranslationMethod=Cartesian  TranslationStandardOffset=10  TranslationLengthUnit=m  TranslationStandardAxis=+Y  TranslationCartesianOffset=bin_pos_offset  TranslationROffset=0  TranslationROffsetUnits=m  TranslationZOffset=0  TranslationZOffsetUnits=m  TranslationThetaOffset=0  TranslationThetaOffsetUnits=deg  RotationMethod=RotationSequence  RotationAngleUnits=deg  RotationStandardAxis=+Z  RotationAngle=90  RotationArbitraryAxis=smiData.RigidTransform(1).axis  FollAlignAxisA=+X  BaseAlignAxisA=+Y  FollAlignAxisB=+Y  BaseAlignAxisB=+Z  RotationSequenceAxes=BaseAxes  RotationSequence=XYZ  RotationSequenceAngles=bin_angle_offset  RotationSequenceAnglesUnits=deg  RotationMatrix=[1 0 0; 0 1 0; 0 0 1]
  Transform5 : sm_lib/Frames and Transforms/Rigid Transform  TranslationMethod=Cartesian  TranslationStandardOffset=10  TranslationLengthUnit=m  TranslationStandardAxis=+Y  TranslationCartesianOffset=chute_pos_offset  TranslationROffset=0  TranslationROffsetUnits=m  TranslationZOffset=0  TranslationZOffsetUnits=m  TranslationThetaOffset=0  TranslationThetaOffsetUnits=deg  RotationMethod=RotationSequence  RotationAngleUnits=deg  RotationStandardAxis=+Z  RotationAngle=90  RotationArbitraryAxis=smiData.RigidTransform(1).axis  FollAlignAxisA=+X  BaseAlignAxisA=+Y  FollAlignAxisB=+Y  BaseAlignAxisB=+Z  RotationSequenceAxes=BaseAxes  RotationSequence=XYZ  RotationSequenceAngles=chute_angle_offset  RotationSequenceAnglesUnits=deg  RotationMatrix=[1 0 0; 0 1 0; 0 0 1]
  bin_1_RIGID1 : Subsystem  Commented=on
  chute2_1_RIGID : Subsystem
  guard_1_RIGID2 : Subsystem
  guard_1_RIGID3 : Subsystem
  shelf_1_RIGID1 : Subsystem
  Transform1 : PMIOPort  Side=Left
  connections:
  Transform2/RConn1 -- guard_1_RIGID2/LConn1
  Transform3/RConn1 -- guard_1_RIGID3/LConn1
  Transform1/RConn1 -- Transform2/LConn1 -- Transform34/LConn1 -- Transform5/LConn1 -- Transform4/LConn1 -- Transform3/LConn1
  bin_1_RIGID1/LConn1 -- Transform4/RConn1
  shelf_1_RIGID1/LConn1 -- Transform34/RConn1
  chute2_1_RIGID/LConn1 -- Transform5/RConn1

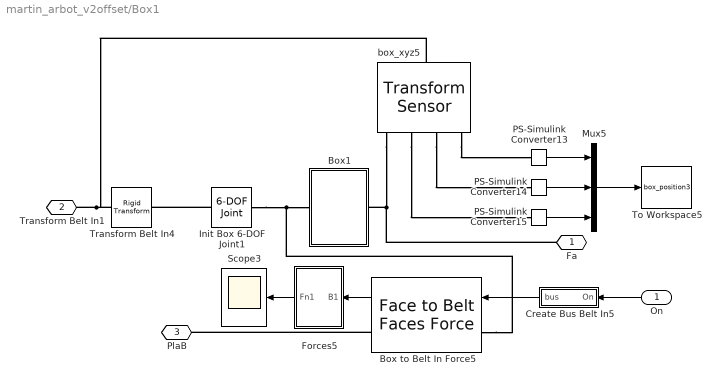
== system martin_arbot_v2offset/Box1 ==
  On : Inport
  Box to Belt In Force5 : Contact_Forces_Lib/3D/Composite Forces/Face to Belt Faces Force  PlaB_x=belt_l  PlaB_y=belt_w  PlaB_z=belt_h/2  FacF_x=cube_d  FacF_y=cube_d  FacF_z=0  FacF_rSph=cube_con_rsph  force_law_pla2pla=Linear  k_contact_pla2pla=1e4  b_contact_pla2pla=1e2  pen_full_damp_F_pla2pla=1e-4  pen_exponent_pla2pla=1  friction_law_pla2pla=Stick-Slip Continuous  mu_kinetic_pla2pla=0.5  mu_static_pla2pla=0.7  v_thr_pla2pla=0.001  vis_on_pla2pla=off  vis_opc_en_box2box=0  vis_len_plaLz=0.0005  vis_clr=[0.9 0.2 0.2]  vis_opc=0.7
      settings: SourceProductName=Simscape Multibody Contact Forces Library
  Box1 : Subsystem  Tag=CustomStyle
  Create Bus Belt In5 : Subsystem
  Forces5 : Subsystem
  Init Box 6-DOF Joint1 : sm_lib/Joints/6-DOF Joint  JointMode=Normal  SenseConstraintForce=off  SenseConstraintForceX=off  SenseConstraintForceY=off  SenseConstraintForceZ=off  SenseConstraintTorque=off  SenseConstraintTorqueX=off  SenseConstraintTorqueY=off  SenseConstraintTorqueZ=off  SenseTotalForce=off  SenseTotalForceX=off  SenseTotalForceY=off  SenseTotalForceZ=off  SenseTotalTorque=off  SenseTotalTorqueX=off  SenseTotalTorqueY=off  SenseTotalTorqueZ=off  CompositeWrenchDir=FollowerOnBase  CompositeWrenchFrame=BaseFrame  PxEquilibriumPosition=0  PxEquilibriumPositionUnits=m  PxSpringStiffness=0  PxSpringStiffnessUnits=N/m  PxDampingCoefficient=0  PxDampingCoefficientUnits=N/(m/s)  PxTorqueActuationMode=NoTorque  PxMotionActuationMode=ComputedMotion  PxSensePosition=off  PxSenseVelocity=off  PxSenseAcceleration=off  PxSenseTorqueForce=off  PxSenseLowerLimitTorqueForce=off  PxSenseUpperLimitTorqueForce=off  PxLowerLimitSpecify=off  PxLowerLimitBound=-1  PxLowerLimitBoundUnits=m  PxLowerLimitStiffness=1e6  PxLowerLimitStiffnessUnits=N/m  PxLowerLimitDamping=1e3  PxLowerLimitDampingUnits=N/(m/s)  PxLowerLimitTransitionRegionWidth=1e-4  PxLowerLimitTransitionRegionWidthUnits=m  PxUpperLimitSpecify=off  PxUpperLimitBound=1  PxUpperLimitBoundUnits=m  PxUpperLimitStiffness=1e6  PxUpperLimitStiffnessUnits=N/m  PxUpperLimitDamping=1e3  PxUpperLimitDampingUnits=N/(m/s)  PxUpperLimitTransitionRegionWidth=1e-4  PxUpperLimitTransitionRegionWidthUnits=m  PxPositionTargetSpecify=off  PxPositionTargetPriority=High  PxPositionTargetValue=0  PxPositionTargetValueUnits=m  PxVelocityTargetSpecify=off  PxVelocityTargetPriority=High  PxVelocityTargetValue=0  PxVelocityTargetValueUnits=m/s  PyEquilibriumPosition=0  PyEquilibriumPositionUnits=m  PySpringStiffness=0  PySpringStiffnessUnits=N/m  PyDampingCoefficient=0  PyDampingCoefficientUnits=N/(m/s)  PyTorqueActuationMode=NoTorque  PyMotionActuationMode=ComputedMotion  PySensePosition=off  PySenseVelocity=off  PySenseAcceleration=off  PySenseTorqueForce=off  PySenseLowerLimitTorqueForce=off  PySenseUpperLimitTorqueForce=off  PyLowerLimitSpecify=off  PyLowerLimitBound=-1  PyLowerLimitBoundUnits=m  PyLowerLimitStiffness=1e6  PyLowerLimitStiffnessUnits=N/m  PyLowerLimitDamping=1e3  PyLowerLimitDampingUnits=N/(m/s)  PyLowerLimitTransitionRegionWidth=1e-4  PyLowerLimitTransitionRegionWidthUnits=m  PyUpperLimitSpecify=off  PyUpperLimitBound=1  PyUpperLimitBoundUnits=m  PyUpperLimitStiffness=1e6  PyUpperLimitStiffnessUnits=N/m  PyUpperLimitDamping=1e3  PyUpperLimitDampingUnits=N/(m/s)  PyUpperLimitTransitionRegionWidth=1e-4  PyUpperLimitTransitionRegionWidthUnits=m  PyPositionTargetSpecify=off  PyPositionTargetPriority=High  PyPositionTargetValue=60e-2  PyPositionTargetValueUnits=m  PyVelocityTargetSpecify=off  PyVelocityTargetPriority=High  PyVelocityTargetValue=0  PyVelocityTargetValueUnits=m/s  PzEquilibriumPosition=0  PzEquilibriumPositionUnits=m  PzSpringStiffness=0  PzSpringStiffnessUnits=N/m  PzDampingCoefficient=0  PzDampingCoefficientUnits=N/(m/s)  PzTorqueActuationMode=NoTorque  PzMotionActuationMode=ComputedMotion  PzSensePosition=off  PzSenseVelocity=off  PzSenseAcceleration=off  PzSenseTorqueForce=off  PzSenseLowerLimitTorqueForce=off  PzSenseUpperLimitTorqueForce=off  PzLowerLimitSpecify=off  PzLowerLimitBound=-1  PzLowerLimitBoundUnits=m  PzLowerLimitStiffness=1e6  PzLowerLimitStiffnessUnits=N/m  PzLowerLimitDamping=1e3  PzLowerLimitDampingUnits=N/(m/s)  PzLowerLimitTransitionRegionWidth=1e-4  PzLowerLimitTransitionRegionWidthUnits=m  PzUpperLimitSpecify=off  PzUpperLimitBound=1  PzUpperLimitBoundUnits=m  PzUpperLimitStiffness=1e6  PzUpperLimitStiffnessUnits=N/m  PzUpperLimitDamping=1e3  PzUpperLimitDampingUnits=N/(m/s)  PzUpperLimitTransitionRegionWidth=1e-4  PzUpperLimitTransitionRegionWidthUnits=m  PzPositionTargetSpecify=on  PzPositionTargetPriority=High  PzPositionTargetValue=(cube_d)/2+0.1  PzPositionTargetValueUnits=m  PzVelocityTargetSpecify=off  PzVelocityTargetPriority=High  PzVelocityTargetValue=0  PzVelocityTargetValueUnits=m/s  SphDefPosRotationMethod=None  SphDefPosRotationAngleUnits=deg  SphDefPosRotationStandardAxis=+Z  SphDefPosRotationAngle=0.0  SphDefPosRotationArbitraryAxis=[0 0 1]  SphDefPosFollAlignAxisA=+X  SphDefPosBaseAlignAxisA=+Y  SphDefPosFollAlignAxisB=+Y  SphDefPosBaseAlignAxisB=+Z  SphDefPosRotationSequenceAxes=FollowerAxes  SphDefPosRotationSequence=XYX  SphDefPosRotationSequenceAngles=[0 0 0]  SphDefPosRotationSequenceAnglesUnits=deg  SphDefPosRotationMatrix=[1 0 0; 0 1 0; 0 0 1]  SphEqPosRotationMethod=None  SphEqPosRotationAngleUnits=deg  SphEqPosRotationStandardAxis=+Z  SphEqPosRotationAngle=0.0  SphEqPosRotationArbitraryAxis=[0 0 1]  SphEqPosFollAlignAxisA=+X  SphEqPosBaseAlignAxisA=+Y  SphEqPosFollAlignAxisB=+Y  SphEqPosBaseAlignAxisB=+Z  SphEqPosRotationSequenceAxes=FollowerAxes  SphEqPosRotationSequence=XYX  SphEqPosRotationSequenceAngles=[0 0 0]  SphEqPosRotationSequenceAnglesUnits=deg  SphEqPosRotationMatrix=[1 0 0; 0 1 0; 0 0 1]  SphSpringStiffness=0  SphSpringStiffnessUnits=N*m/deg  SphDampingCoefficient=0  SphDampingCoefficientUnits=N*m/(deg/s)  SphActuateTorqueX=off  SphActuateTorqueY=off  SphActuateTorqueZ=off  SphActuateTorque=off  SphTorqueActuationMode=NoTorque  SphMotionActuationMode=ComputedMotion  SphActuationFrame=BaseFrame  SphSensePosition=off  SphSenseVelocityX=off  SphSenseVelocityY=off  SphSenseVelocityZ=off  SphSenseVelocity=off  SphSenseAccelerationX=off  SphSenseAccelerationY=off  SphSenseAccelerationZ=off  SphSenseAcceleration=off  SphSenseTorqueX=off  SphSenseTorqueY=off  SphSenseTorqueZ=off  SphSenseTorqueForce=off  SphSenseLowerLimitTorqueMag=off  SphSenseUpperLimitTorqueMag=off  SphSensingFrame=BaseFrame  SphLowerLimitSpecify=off  SphLowerLimitBound=15  SphLowerLimitBoundUnits=deg  SphLowerLimitStiffness=1e4  SphLowerLimitStiffnessUnits=N*m/deg  SphLowerLimitDamping=10  SphLowerLimitDampingUnits=N*m/(deg/s)  SphLowerLimitTransitionRegionWidth=0.1  SphLowerLimitTransitionRegionWidthUnits=deg  SphUpperLimitSpecify=off  SphUpperLimitBound=45  SphUpperLimitBoundUnits=deg  SphUpperLimitStiffness=1e4  SphUpperLimitStiffnessUnits=N*m/deg  SphUpperLimitDamping=10  SphUpperLimitDampingUnits=N*m/(deg/s)  SphUpperLimitTransitionRegionWidth=0.1  SphUpperLimitTransitionRegionWidthUnits=deg  SphPositionTargetRotationMethod=RotationSequence  SphPositionTargetRotationAngleUnits=deg  SphPositionTargetRotationStandardAxis=+X  SphPositionTargetRotationAngle=0+180  SphPositionTargetRotationArbitraryAxis=[0 0 1]  SphPositionTargetFollAlignAxisA=+X  SphPositionTargetBaseAlignAxisA=+Y  SphPositionTargetFollAlignAxisB=+Y  SphPositionTargetBaseAlignAxisB=+Z  SphPositionTargetRotationSequenceAxes=FollowerAxes  SphPositionTargetRotationSequence=XZX  SphPositionTargetRotationSequenceAngles=[180 10 0]  SphPositionTargetRotationSequenceAnglesUnits=deg  SphPositionTargetRotationMatrix=[1 0 0; 0 1 0; 0 0 1]  SphPositionTargetSpecify=on  SphPositionTargetPriority=High  SphVelocityTargetValue=[0 0 0]  SphVelocityTargetValueUnits=deg/s  SphVelocityTargetSpecify=off  SphVelocityTargetPriority=High  SphVelocityTargetInFollowerFrame=on
  Mux5 : Mux  Inputs=3
  PS-Simulink Converter13 : nesl_utility/PS-Simulink Converter  PhysicalDomain=network_engine_domain  SubClassName=ps_output  LeftPortType=input  RightPortType=output  PseudoPeriodic=off  Frequencies=[]  Unit=m  AffineConversion=off
  PS-Simulink Converter14 : nesl_utility/PS-Simulink Converter  PhysicalDomain=network_engine_domain  SubClassName=ps_output  LeftPortType=input  RightPortType=output  PseudoPeriodic=off  Frequencies=[]  Unit=m  AffineConversion=off
  PS-Simulink Converter15 : nesl_utility/PS-Simulink Converter  PhysicalDomain=network_engine_domain  SubClassName=ps_output  LeftPortType=input  RightPortType=output  PseudoPeriodic=off  Frequencies=[]  Unit=m  AffineConversion=off
  Scope3 : Scope
  To Workspace5 : ToWorkspace  VariableName=box_position3  SaveFormat=Structure With Time  SampleTime=0.001
  Transform Belt In4 : sm_lib/Frames and Transforms/Rigid Transform  TranslationMethod=Cartesian  TranslationStandardOffset=0  TranslationLengthUnit=m  TranslationStandardAxis=+Y  TranslationCartesianOffset=box1_pos_offset  TranslationROffset=0  TranslationROffsetUnits=m  TranslationZOffset=0  TranslationZOffsetUnits=m  TranslationThetaOffset=0  TranslationThetaOffsetUnits=deg  RotationMethod=None  RotationAngleUnits=deg  RotationStandardAxis=+Z  RotationAngle=-90  RotationArbitraryAxis=[0 0 1]  FollAlignAxisA=+X  BaseAlignAxisA=+Y  FollAlignAxisB=+Y  BaseAlignAxisB=+Z  RotationSequenceAxes=FollowerAxes  RotationSequence=XYZ  RotationSequenceAngles=box_angle_offset  RotationSequenceAnglesUnits=deg  RotationMatrix=[1 0 0; 0 1 0; 0 0 1]
  box_xyz5 : sm_lib/Frames and Transforms/Transform Sensor  MeasurementFrame=Base  SenseAngle=off  SenseAxis=off  SenseAngle1=off  SenseAngle2=off  SenseAngle3=off  SenseQ=off  SenseR=off  SenseOmegaX=off  SenseOmegaY=off  SenseOmegaZ=off  SenseOmega1=off  SenseOmega2=off  SenseOmega3=off  SenseQDot=off  SenseRDot=off  SenseAlphaX=off  SenseAlphaY=off  SenseAlphaZ=off  SenseAlpha1=off  SenseAlpha2=off  SenseAlpha3=off  SenseQDDot=off  SenseRDDot=off  SenseX=on  SenseY=on  SenseZ=on  SenseRad=off  SenseAzim=off  SenseDist=off  SenseInc=off  SenseXDot=off  SenseYDot=off  SenseZDot=off  SenseRadDot=off  SenseAzimDot=off  SenseDistDot=off  SenseIncDot=off  SenseXDDot=off  SenseYDDot=off  SenseZDDot=off  SenseRadDDot=off  SenseAzimDDot=off  SenseDistDDot=off  SenseIncDDot=off
  Fa : PMIOPort  Side=Right
  Transform Belt In1 : PMIOPort  Port=2  Side=Left
  PlaB : PMIOPort  Port=3  Side=Right
  wires:
  PS-Simulink Converter13/1 -> Mux5/1
  Forces5/1(Fn1) -> Scope3/1
  PS-Simulink Converter14/1 -> Mux5/2
  PS-Simulink Converter15/1 -> Mux5/3
  Mux5/1 -> To Workspace5/1
  Box to Belt In Force5/1 -> Forces5/1(B1)
  On/1 -> Create Bus Belt In5/1(On)
  Create Bus Belt In5/1(bus) -> Box to Belt In Force5/1
  connections:
  box_xyz5/RConn1 -- Box1/RConn1 -- Fa/RConn1
  box_xyz5/RConn2 -- PS-Simulink Converter15/LConn1
  box_xyz5/RConn3 -- PS-Simulink Converter14/LConn1
  box_xyz5/RConn4 -- PS-Simulink Converter13/LConn1
  Box to Belt In Force5/LConn1 -- Init Box 6-DOF Joint1/RConn1 -- Box1/LConn1
  Init Box 6-DOF Joint1/LConn1 -- Transform Belt In4/RConn1
  Box to Belt In Force5/RConn1 -- PlaB/RConn1
  Transform Belt In4/LConn1 -- box_xyz5/LConn1 -- Transform Belt In1/RConn1
